simulink subsystem "DecelerationMaking"  (R2022b)
settings: Solver=VariableStepAuto  StartTime=0.0  StopTime=10.0  RelTol=1e-3
libraries: simulink x1
settings Model: Creator=hubkapatrik  LastModifiedBy=hubkapatrik

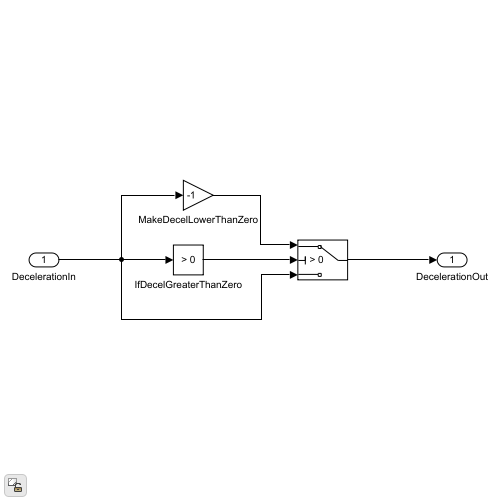
[thumbnail: Simulink's stored preview of the top-level diagram]
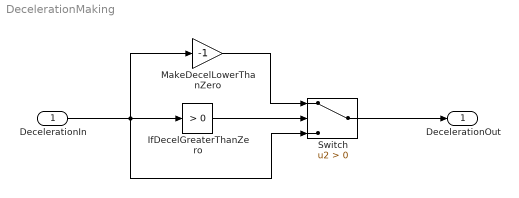
== system DecelerationMaking ==
  DecelerationIn : Inport
  IfDecelGreaterThanZero : simulink/Logic and Bit Operations/Compare To Constant  relop=>  const=0  OutDataTypeStr=boolean
  MakeDecelLowerThanZero : Gain  Gain=-1
  Switch : Switch  Criteria=u2 > Threshold  SaturateOnIntegerOverflow=off  InputSameDT=off
  DecelerationOut : Outport
  wires:
  Switch/1 -> DecelerationOut/1
  IfDecelGreaterThanZero/1 -> Switch/2
  DecelerationIn/1 -> IfDecelGreaterThanZero/1, Switch/3, MakeDecelLowerThanZero/1
  MakeDecelLowerThanZero/1 -> Switch/1
